simulink model "RunFlexionExtension2024a"  (R2024a)
settings: Solver=VariableStepAuto  StartTime=0.0  StopTime=Inf  RelTol=1e-3
libraries: instrumentseriallib x2
settings Model: Creator=roman  LastModifiedBy=roman
settings ConfigComp: CovBoundaryAbsTol=1.0e-5

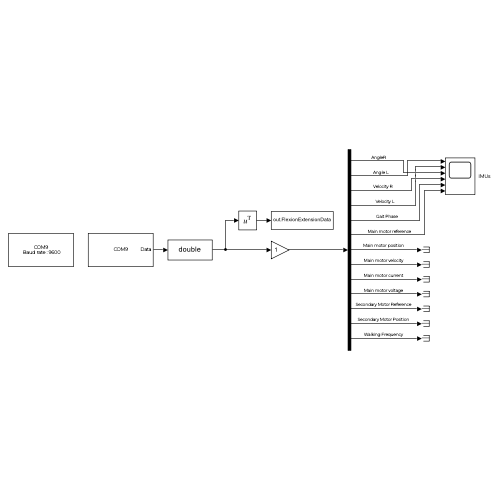
[thumbnail: Simulink's stored preview of the top-level diagram]
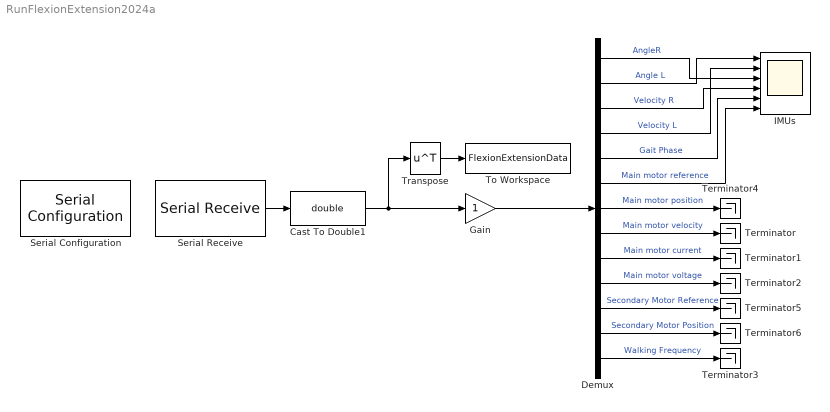
== system RunFlexionExtension2024a ==
  Cast To Double1 : DataTypeConversion  OutDataTypeStr=double  SaturateOnIntegerOverflow=off  RndMeth=Floor
  Demux : Demux  Outputs=13
  Gain : Gain
  IMUs : Scope  NumInputPorts=6
  Serial Configuration : instrumentseriallib/Serial Configuration  Priority=-200000  PortSel=COM9  Port=COM9  ComPort=COM9  BaudRate=9600  DataBits=8  Parity=none  StopBits=1  ByteOrder=little-endian  FlowControl=none  Timeout=10  SimulateUsing=Interpreted execution  BlockInModel=on  aMode=1
      settings: LibrarySourceBlock=embeddedtargetslib/Host Communication/Serial Configuration
  Serial Receive : instrumentseriallib/Serial Receive  Priority=1  PortSel=COM9  Port=COM9  ComPort=COM9  DataType=double  SaveDataType=uint8  ToggleHeader=off  Header=[]  ToggleDataSize=on  DataSize=13  ToggleTerminator=off  Terminator=<none>  CustomTerminator=[]  InputFormat=Column major  EnableBlockingMode=on  ActionDataUnavailable=Output last received value  ActionWhenDataUnavailable=Output last received value  CustomValue=0  SampleTime=0.01  SimulateUsing=Interpreted execution  BlockInModel=on  aMode=1
      settings: LibrarySourceBlock=embeddedtargetslib/Host Communication/Serial Receive
  Terminator{,1..6} (7 alike) : Terminator
  To Workspace : ToWorkspace  VariableName=FlexionExtensionData  SampleTime=-1
      settings: Save2DSignal=2-D array (concatenate along first dimension)
  Transpose : Math  Operator=transpose
  wires:
  Serial Receive/1 -> Cast To Double1/1
  Cast To Double1/1 -> Gain/1, Transpose/1
  Transpose/1 -> To Workspace/1
  Gain/1 -> Demux/1
  Demux/1 -> IMUs/3  "AngleR"
  Demux/2 -> IMUs/1  "Angle L"
  Demux/3 -> IMUs/4  "Velocity R"
  Demux/4 -> IMUs/2  "Velocity L"
  Demux/11 -> Terminator5/1  "Secondary Motor Reference"
  Demux/12 -> Terminator6/1  "Secondary Motor Position"
  Demux/5 -> IMUs/5  "Gait Phase"
  Demux/6 -> IMUs/6  "Main motor reference"
  Demux/7 -> Terminator4/1  "Main motor position"
  Demux/8 -> Terminator/1  "Main motor velocity"
  Demux/9 -> Terminator1/1  "Main motor current"
  Demux/10 -> Terminator2/1  "Main motor voltage"
  Demux/13 -> Terminator3/1  "Walking Frequency"
